simulink model "trimLiepke"  (R2021a)
settings: Solver=ode45  StartTime=0.0  StopTime=1000  RelTol=1e-3  EnableMultiTasking=on
undefined symbols (not defined in the file or in its folder): alpha_matrix, alphai, alt_matrix, b, beta, cbar, CD_0, CD_alpha, CD_de, CD_ih, CD_q, CL_0, Cl_0, CL_alpha, Cl_beta, Cl_da, CL_de, Cl_dr, CL_ih, Cl_p, CL_q, Cl_r, cla_matrix, clb_matrix, clp_matrix, clq_matrix, clr_matrix, Cm_0, Cm_alpha, Cm_de, Cm_ih, Cm_q, cma_matrix, cmq_matrix, Cn_0, Cn_beta, Cn_da, Cn_dr, Cn_p, Cn_r, cnb_matrix, cnp_matrix, cnr_matrix, CY_0, CY_beta, CY_da, CY_dr, CY_p, CY_r, cyb_matrix, cyp_matrix, H, Ix, Iy, Iz, Jxy, Jxz, Jyz, m, mach_matrix ... (+10)
libraries: airlib x3
(part 2 of 2)

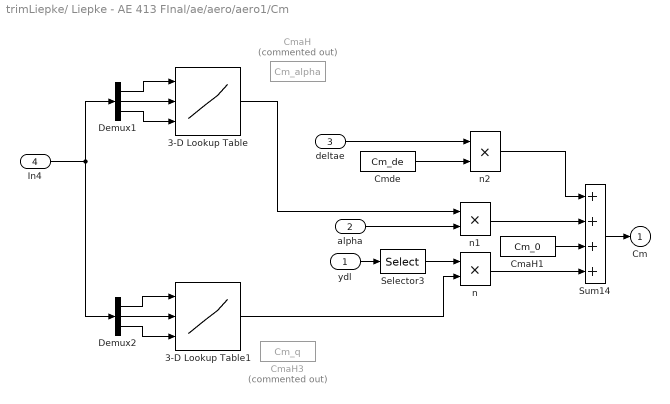
== system trimLiepke/ Liepke - AE 413 FInal/ae/aero/aero1/Cm ==
  ydl : Inport
  alpha : Inport  Port=2
  deltae : Inport  Port=3
  In4 : Inport  Port=4
  3-D Lookup Table : Lookup_n-D  NumberOfTableDimensions=3  BreakpointsForDimension1=alpha_matrix  BreakpointsForDimension2=mach_matrix  BreakpointsForDimension3=alt_matrix  Table=cma_matrix  InternalRulePriority=Speed  RndMeth=Simplest  InputSameDT=on
      settings: InputPortMap=u0,u1,u2
  3-D Lookup Table1 : Lookup_n-D  NumberOfTableDimensions=3  BreakpointsForDimension1=alpha_matrix  BreakpointsForDimension2=mach_matrix  BreakpointsForDimension3=alt_matrix  Table=cmq_matrix  InternalRulePriority=Speed  RndMeth=Simplest  InputSameDT=on
      settings: InputPortMap=u0,u1,u2
  CmaH : Constant  Commented=on  Value=Cm_alpha
  CmaH1 : Constant  Value=Cm_0
  CmaH3 : Constant  Commented=on  Value=Cm_q
  Cmde : Constant  Value=Cm_de
  Demux1 : Demux  Outputs=3
  Demux2 : Demux  Outputs=3
  Selector3 : Selector  InputPortWidth=3  IndexOptions=Index vector (dialog)  Indices=[2]  OutputSizes=1
  Sum14 : Sum  Inputs=++++  InputSameDT=on  SaturateOnIntegerOverflow=on  OutDataTypeStr=Inherit: Same as first input
  n : Product  InputSameDT=on  SaturateOnIntegerOverflow=on  OutDataTypeStr=Inherit: Same as first input
  n1 : Product  InputSameDT=on  SaturateOnIntegerOverflow=on  OutDataTypeStr=Inherit: Same as first input
  n2 : Product  InputSameDT=on  SaturateOnIntegerOverflow=on  OutDataTypeStr=Inherit: Same as first input
  Cm : Outport  VectorParamsAs1DForOutWhenUnconnected=off
  wires:
  Selector3/1 -> n/1
  n1/1 -> Sum14/2
  ydl/1 -> Selector3/1
  n/1 -> Sum14/4
  Sum14/1 -> Cm/1
  CmaH1/1 -> Sum14/3
  alpha/1 -> n1/2
  Cmde/1 -> n2/2
  n2/1 -> Sum14/1
  deltae/1 -> n2/1
  Demux1/2 -> 3-D Lookup Table/2
  Demux1/3 -> 3-D Lookup Table/3
  Demux1/1 -> 3-D Lookup Table/1
  Demux2/1 -> 3-D Lookup Table1/1
  Demux2/3 -> 3-D Lookup Table1/3
  Demux2/2 -> 3-D Lookup Table1/2
  In4/1 -> Demux1/1, Demux2/1
  3-D Lookup Table/1 -> n1/1
  3-D Lookup Table1/1 -> n/2

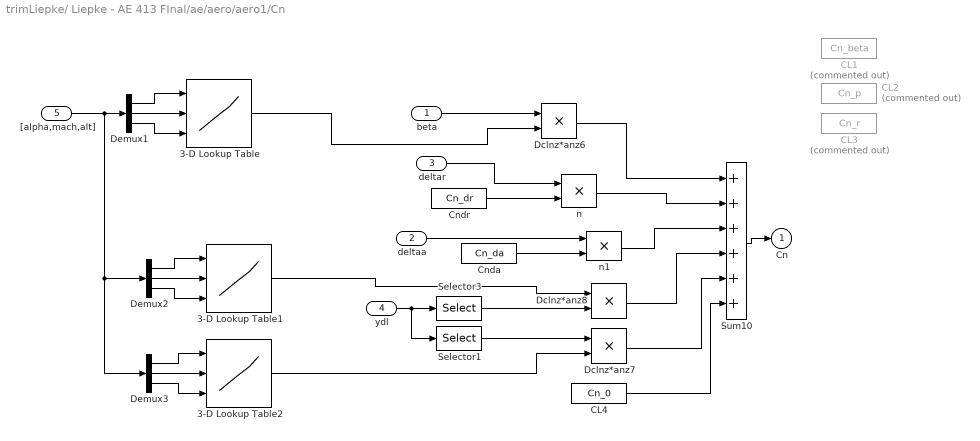
== system trimLiepke/ Liepke - AE 413 FInal/ae/aero/aero1/Cn ==
  beta : Inport
  deltaa : Inport  Port=2
  deltar : Inport  Port=3
  ydl : Inport  Port=4
  "[alpha,mach,alt]" : Inport  Port=5
  3-D Lookup Table : Lookup_n-D  NumberOfTableDimensions=3  BreakpointsForDimension1=alpha_matrix  BreakpointsForDimension2=mach_matrix  BreakpointsForDimension3=alt_matrix  Table=cnb_matrix  InternalRulePriority=Speed  RndMeth=Simplest  InputSameDT=on
      settings: InputPortMap=u0,u1,u2
  3-D Lookup Table1 : Lookup_n-D  NumberOfTableDimensions=3  BreakpointsForDimension1=alpha_matrix  BreakpointsForDimension2=mach_matrix  BreakpointsForDimension3=alt_matrix  Table=cnp_matrix  InternalRulePriority=Speed  RndMeth=Simplest  InputSameDT=on
      settings: InputPortMap=u0,u1,u2
  3-D Lookup Table2 : Lookup_n-D  NumberOfTableDimensions=3  BreakpointsForDimension1=alpha_matrix  BreakpointsForDimension2=mach_matrix  BreakpointsForDimension3=alt_matrix  Table=cnr_matrix  InternalRulePriority=Speed  RndMeth=Simplest  InputSameDT=on
      settings: InputPortMap=u0,u1,u2
  CL1 : Constant  Commented=on  Value=Cn_beta  SampleTime=-1
  CL2 : Constant  Commented=on  Value=Cn_p
  CL3 : Constant  Commented=on  Value=Cn_r
  CL4 : Constant  Value=Cn_0  SampleTime=-1
  Cnda : Constant  Value=Cn_da  SampleTime=-1
  Cndr : Constant  Value=Cn_dr  SampleTime=-1
  Dclnz*anz6 : Product  InputSameDT=on  SaturateOnIntegerOverflow=on  OutDataTypeStr=Inherit: Same as first input
  Dclnz*anz7 : Product  InputSameDT=on  SaturateOnIntegerOverflow=on  OutDataTypeStr=Inherit: Same as first input
  Dclnz*anz8 : Product  InputSameDT=on  SaturateOnIntegerOverflow=on  OutDataTypeStr=Inherit: Same as first input
  Demux1 : Demux  Outputs=3
  Demux2 : Demux  Outputs=3
  Demux3 : Demux  Outputs=3
  Selector1 : Selector  InputPortWidth=3  IndexOptions=Index vector (dialog)  Indices=[3]  OutputSizes=1
  Selector3 : Selector  InputPortWidth=3  IndexOptions=Index vector (dialog)  Indices=[1]  OutputSizes=1
  Sum10 : Sum  Inputs=6  InputSameDT=on  SaturateOnIntegerOverflow=on  OutDataTypeStr=Inherit: Same as first input
  n : Product  InputSameDT=on  SaturateOnIntegerOverflow=on  OutDataTypeStr=Inherit: Same as first input
  n1 : Product  InputSameDT=on  SaturateOnIntegerOverflow=on  OutDataTypeStr=Inherit: Same as first input
  Cn : Outport  VectorParamsAs1DForOutWhenUnconnected=off
  wires:
  beta/1 -> Dclnz*anz6/1
  Selector3/1 -> Dclnz*anz8/2
  Selector1/1 -> Dclnz*anz7/1
  3-D Lookup Table2/1 -> Dclnz*anz7/2
  ydl/1 -> Selector3/1, Selector1/1
  Dclnz*anz6/1 -> Sum10/1
  3-D Lookup Table1/1 -> Dclnz*anz8/1
  Sum10/1 -> Cn/1
  Dclnz*anz8/1 -> Sum10/4
  Dclnz*anz7/1 -> Sum10/5
  n1/1 -> Sum10/3
  deltar/1 -> n/1
  Cndr/1 -> n/2
  n/1 -> Sum10/2
  Cnda/1 -> n1/2
  deltaa/1 -> n1/1
  CL4/1 -> Sum10/6
  Demux1/1 -> 3-D Lookup Table/1
  Demux1/3 -> 3-D Lookup Table/3
  Demux1/2 -> 3-D Lookup Table/2
  3-D Lookup Table/1 -> Dclnz*anz6/2
  Demux2/1 -> 3-D Lookup Table1/1
  Demux2/3 -> 3-D Lookup Table1/3
  Demux2/2 -> 3-D Lookup Table1/2
  Demux3/2 -> 3-D Lookup Table2/2
  "[alpha,mach,alt]"/1 -> Demux3/1, Demux2/1, Demux1/1
  Demux3/1 -> 3-D Lookup Table2/1
  Demux3/3 -> 3-D Lookup Table2/3

== system trimLiepke/ Liepke - AE 413 FInal/ae/aero/aero1/Stability 2 Body Axis ==
  alpha : Inport
  FsMb : Inport  Port=2
  Demux2 : Demux  Outputs=3
      settings: DisplayOption=none
  Mux1 : Mux  Inputs=3
  Product{2..5} (4 alike) : Product  InputSameDT=on  RndMeth=Zero  SaturateOnIntegerOverflow=on  OutDataTypeStr=Inherit: Same as first input
  Sum3 : Sum  Inputs=-+  InputSameDT=on  SaturateOnIntegerOverflow=on  OutDataTypeStr=Inherit: Same as first input
  Sum4 : Sum  Inputs=--  InputSameDT=on  SaturateOnIntegerOverflow=on  OutDataTypeStr=Inherit: Same as first input
  cos alpha : Fcn  Expr=cos(u[1])
  sin alpha : Fcn
  FbMb : Outport  VectorParamsAs1DForOutWhenUnconnected=off
  wires:
  Demux2/2 -> Mux1/2
  cos alpha/1 -> Product2/1, Product5/1
  Demux2/1 -> Product2/2, Product4/2
  Product2/1 -> Sum3/1
  Product3/1 -> Sum3/2
  Sum3/1 -> Mux1/1
  sin alpha/1 -> Product3/1, Product4/1
  Demux2/3 -> Product3/2, Product5/2
  Product4/1 -> Sum4/1
  Product5/1 -> Sum4/2
  Sum4/1 -> Mux1/3
  alpha/1 -> sin alpha/1, cos alpha/1
  Mux1/1 -> FbMb/1
  FsMb/1 -> Demux2/1

== system trimLiepke/ Liepke - AE 413 FInal/eqm/ODE/Eulerdot/0 ==

== system trimLiepke/ Liepke - AE 413 FInal/eqm/ODE/Vabdot/0 ==

== system trimLiepke/ Liepke - AE 413 FInal/eqm/ODE/pqrdot/0 ==

== system trimLiepke/ Liepke - AE 413 FInal/eqm/ODE/pqrdot/GM2  ==
  In1 : Inport
  Matrix Gain : StateSpace  A=[]  B=[]  C=[]  D=M  InitialCondition=0
  Out1 : Outport
  wires:
  In1/1 -> Matrix Gain/1
  Matrix Gain/1 -> Out1/1

== system trimLiepke/ Liepke - AE 413 FInal/eqm/ODE/xyHdot/0 ==
